simulink model "kkadai14"  (R2021b)
settings: Solver=VariableStepAuto  StartTime=0.0  StopTime=500  RelTol=1e-3
settings Model: Creator=tomotomo  LastModifiedBy=tomotomo

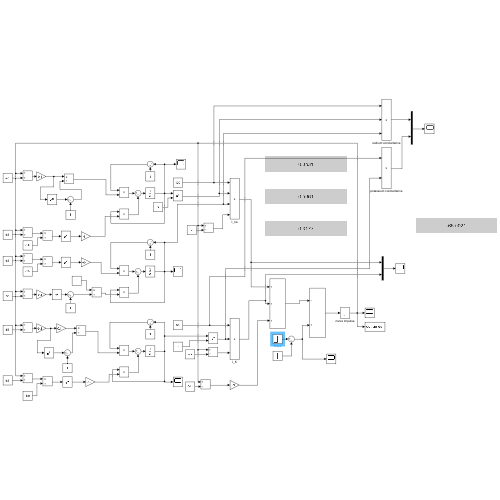
[thumbnail: Simulink's stored preview of the top-level diagram]
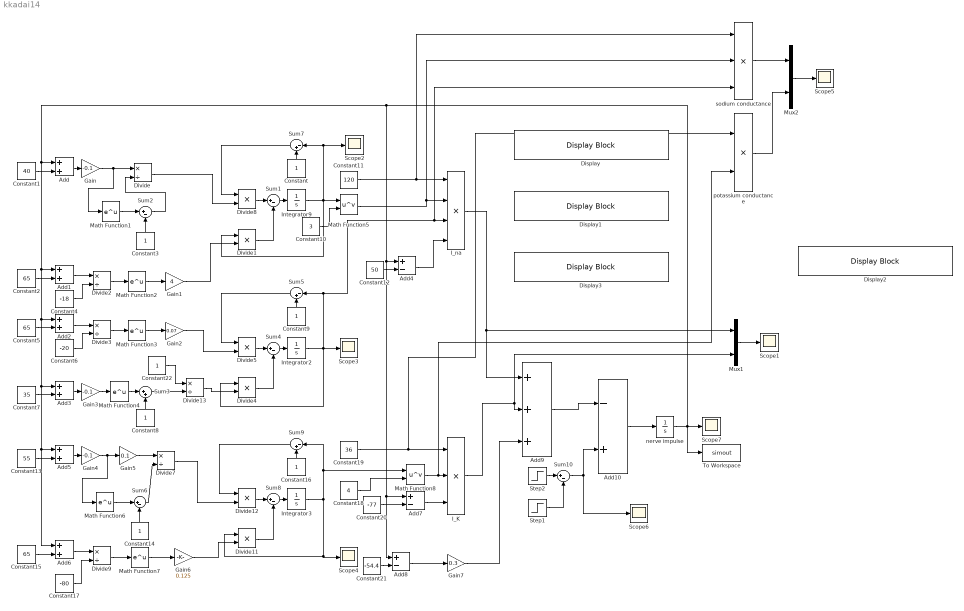
== system kkadai14 ==
  Add{,1..3,5..6} (6 alike) : Sum
  Add10 : Sum  Inputs=-+
  Add4 : Sum  Inputs=+-
  Add7 : Sum  Inputs=+-
  Add8 : Sum  Inputs=+-
  Add9 : Sum  Inputs=+++
  Constant{,3,8..9,14,16,22} (7 alike) : Constant
  Constant1 : Constant  Value=40
  Constant10 : Constant  Value=3
  Constant11 : Constant  Value=120
  Constant12 : Constant  Value=50
  Constant13 : Constant  Value=55
  Constant15 : Constant  Value=65
  Constant17 : Constant  Value=-80
  Constant18 : Constant  Value=4
  Constant19 : Constant  Value=36
  Constant2 : Constant  Value=65
  Constant20 : Constant  Value=-77
  Constant21 : Constant  Value=-54.4
  Constant4 : Constant  Value=-18
  Constant5 : Constant  Value=65
  Constant6 : Constant  Value=-20
  Constant7 : Constant  Value=35
  Display{,1..3} (4 alike) : DisplayBlock  LabelPosition=Hide  Format=short  Transparency=1
  Divide{,2..3,7,9,13} (6 alike) : Product  Inputs=*/
  Divide{1,4..5,8,11..12} (6 alike) : Product  Inputs=**
  Gain : Gain  Gain=-0.1
  Gain1 : Gain  Gain=4
  Gain2 : Gain  Gain=0.07
  Gain3 : Gain  Gain=-0.1
  Gain4 : Gain  Gain=-0.1
  Gain5 : Gain  Gain=0.1
  Gain6 : Gain  Gain=0.125
  Gain7 : Gain  Gain=0.3
  I_K : Product  Inputs=***
  I_na : Product  Inputs=****
  Integrator2 : Integrator  InitialCondition=0.5961
  Integrator3 : Integrator  InitialCondition=0.3177
  Integrator9 : Integrator  InitialCondition=0.0529
  Math Function{1..4,6..7} (6 alike) : Math  SaturateOnIntegerOverflow=on
  Math Function5 : Math  Operator=pow  SaturateOnIntegerOverflow=on
  Math Function8 : Math  Operator=pow  SaturateOnIntegerOverflow=on
  Mux1 : Mux  Inputs=2
  Mux2 : Mux  Inputs=2
  Scope{1..7} (7 alike) : Scope
  Step1 : Step  Time=450  After=11.5  SampleTime=0
  Step2 : Step  Time=50  After=11.5  SampleTime=0
  Sum{1..2,4,6,8,10} (6 alike) : Sum  Inputs=|+-
  Sum3 : Sum  Inputs=|++
  Sum5 : Sum  Inputs=|-+
  Sum7 : Sum  Inputs=|-+
  Sum9 : Sum  Inputs=|-+
  To Workspace : ToWorkspace  VariableName=simout  SaveFormat=Timeseries  SampleTime=-1
  nerve impulse : Integrator  InitialCondition=-65
  potassium conductance : Product  Inputs=**
  sodium conductance : Product  Inputs=***
  wires:
  Constant13/1 -> Add5/2
  Sum10/1 -> Scope6/1, Add10/2
  Constant7/1 -> Add3/2
  potassium conductance/1 -> Mux2/2
  Divide3/1 -> Math Function3/1
  Add10/1 -> nerve impulse/1
  Add5/1 -> Gain4/1
  Math Function4/1 -> Sum3/1
  Gain2/1 -> Divide5/2
  Add4/1 -> I_na/4
  nerve impulse/1 -> Scope7/1, To Workspace/1, Add8/1, Add7/1, Add4/1, Add6/1, Add5/1, Add3/1, Add2/1, Add1/1, Add/1
  Gain/1 -> Divide/1, Math Function1/1
  Step1/1 -> Sum10/2
  Divide9/1 -> Math Function7/1
  Math Function7/1 -> Gain6/1
  Add3/1 -> Gain3/1
  Constant16/1 -> Sum9/2
  Sum4/1 -> Integrator2/1
  Constant2/1 -> Add1/2
  Math Function8/1 -> potassium conductance/2, I_K/2
  Gain4/1 -> Gain5/1, Math Function6/1
  Add9/1 -> Add10/1
  Add8/1 -> Gain7/1
  Divide12/1 -> Sum8/1
  Gain3/1 -> Math Function4/1
  Constant12/1 -> Add4/2
  Sum5/1 -> Divide5/1
  Constant17/1 -> Divide9/2
  Add6/1 -> Divide9/1
  Math Function5/1 -> sodium conductance/2, I_na/2
  Divide5/1 -> Sum4/1
  Gain7/1 -> Add9/3
  Math Function2/1 -> Gain1/1
  Constant18/1 -> Math Function8/2
  Gain5/1 -> Divide7/1
  Sum6/1 -> Divide7/2
  Constant15/1 -> Add6/2
  Gain6/1 -> Divide11/2
  Sum9/1 -> Divide12/1
  Divide8/1 -> Sum1/1
  Sum7/1 -> Divide8/1
  Sum1/1 -> Integrator9/1
  Constant5/1 -> Add2/2
  Constant3/1 -> Sum2/2
  Integrator3/1 -> Divide11/1, Scope4/1, Sum9/1, Math Function8/1
  Integrator2/1 -> Scope3/1, Sum5/1, sodium conductance/3, I_na/3, Divide4/1
  Sum8/1 -> Integrator3/1
  Add/1 -> Gain/1
  Math Function6/1 -> Sum6/1
  Math Function1/1 -> Sum2/1
  I_na/1 -> Add9/1, Mux1/1
  Add1/1 -> Divide2/1
  Constant10/1 -> Math Function5/2
  Divide2/1 -> Math Function2/1
  Constant21/1 -> Add8/2
  Constant/1 -> Sum7/2
  Constant4/1 -> Divide2/2
  Integrator9/1 -> Divide1/1, Math Function5/1, Scope2/1, Sum7/1
  Divide/1 -> Divide8/2
  Constant9/1 -> Sum5/2
  Divide4/1 -> Sum4/2
  Constant1/1 -> Add/2
  Constant11/1 -> I_na/1, sodium conductance/1
  Step2/1 -> Sum10/1
  Constant6/1 -> Divide3/2
  Gain1/1 -> Divide1/2
  Sum2/1 -> Divide/2
  Constant14/1 -> Sum6/2
  Constant20/1 -> Add7/2
  Divide1/1 -> Sum1/2
  Divide7/1 -> Divide12/2
  I_K/1 -> Mux1/2, Add9/2
  Add7/1 -> I_K/3
  Constant19/1 -> potassium conductance/1, I_K/1
  Mux1/1 -> Scope1/1
  sodium conductance/1 -> Mux2/1
  Divide13/1 -> Divide4/2
  Divide11/1 -> Sum8/2
  Constant22/1 -> Divide13/1
  Math Function3/1 -> Gain2/1
  Sum3/1 -> Divide13/2
  Mux2/1 -> Scope5/1
  Add2/1 -> Divide3/1
  Constant8/1 -> Sum3/2
